simulink model "propagatorN"  (R2019b)
settings: Solver=ode113  StartTime=0.0  StopTime=86400  MaxStep=0.05  MinStep=1e-4  RelTol=1e-3  AbsTol=1e-13
values from neighbouring files (symbols this model uses):
  C = zeros(lmax,lmax)    [INIT.m]    (also in trajGen.m)
  J = zeros(lmax,1)    [INIT.m]    (also in trajGen.m)
  mi = 398600.435507    [INIT.m]    (also in trajGen.m)
  Rp = 6371    [INIT.m]    (also in trajGen.m)
  S = zeros(lmax,lmax)    [INIT.m]    (also in trajGen.m)
  X0 = [ R0 ; V0 ]    [INIT.m]    (also in trajGen.m)
settings Model: SimulationMode=rapid-accelerator  Creator=tomma  LastModifiedBy=antoniogenova

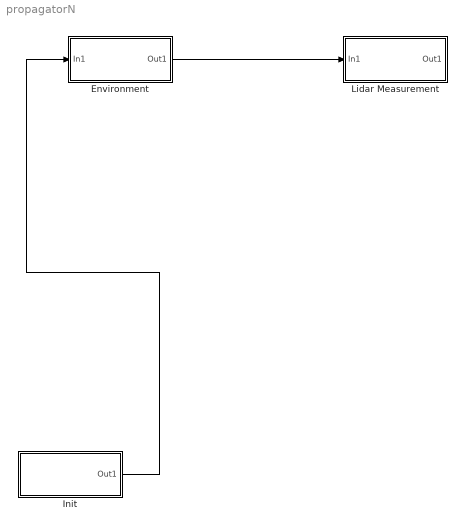
== system propagatorN ==
  "Environment " : Subsystem
  "Init " : Subsystem
  Lidar Measurement : Subsystem
  wires:
  "Init "/1(Out1) -> "Environment "/1(In1)
  "Environment "/1(Out1) -> Lidar Measurement/1(In1)

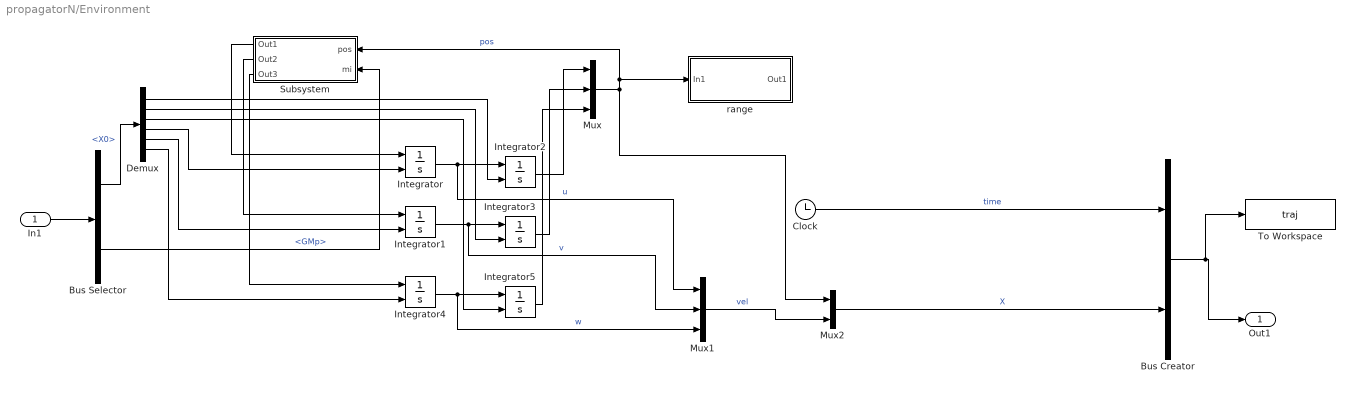
== system propagatorN/Environment  ==
  In1 : Inport
  Bus Creator : BusCreator  Inputs=2
  Bus Selector : BusSelector  OutputSignals=X0,GMp
  Clock : Clock
  Demux : Demux  Outputs=6
  Integrator{,1..5} (6 alike) : Integrator  InitialConditionSource=external  ContinuousStateAttributes="\"\""
  Mux : Mux  Inputs=3
  Mux1 : Mux  Inputs=3
  Mux2 : Mux  Inputs=2
  Subsystem : Subsystem
  To Workspace : ToWorkspace  VariableName=traj  SaveFormat=Timeseries  SampleTime=-1
  range : Subsystem
  Out1 : Outport
  wires:
  In1/1 -> Bus Selector/1
  Integrator4/1 -> Mux1/3, Integrator5/1  "w"
  Integrator1/1 -> Mux1/2, Integrator3/1  "v"
  Integrator/1 -> Mux1/1, Integrator2/1  "u"
  Bus Selector/1 -> Demux/1  "<X0>"
  Mux/1 -> Mux2/1, Subsystem/1(pos), range/1(In1)  "pos"
  Subsystem/1(Out1) -> Integrator/1
  Subsystem/2(Out2) -> Integrator1/1
  Subsystem/3(Out3) -> Integrator4/1
  Integrator2/1 -> Mux/1
  Integrator3/1 -> Mux/2
  Integrator5/1 -> Mux/3
  Mux1/1 -> Mux2/2  "vel"
  Bus Creator/1 -> To Workspace/1, Out1/1
  Bus Selector/2 -> Subsystem/2(mi)  "<GMp>"
  Demux/2 -> Integrator3/2
  Demux/1 -> Integrator2/2
  Demux/3 -> Integrator5/2
  Demux/4 -> Integrator/2
  Demux/5 -> Integrator1/2
  Demux/6 -> Integrator4/2
  Clock/1 -> Bus Creator/1  "time"
  Mux2/1 -> Bus Creator/2  "X"

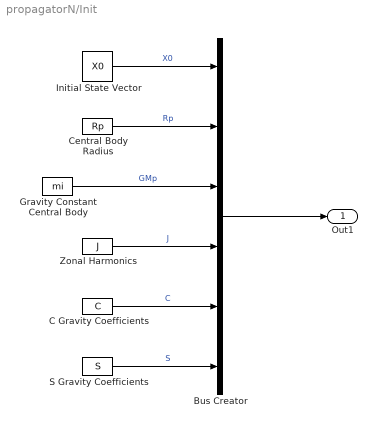
== system propagatorN/Init  ==
  Bus Creator : BusCreator  Inputs=6
  C Gravity Coefficients : Constant  Value=C
  Central Body Radius : Constant  Value=Rp
  Gravity Constant Central Body : Constant  Value=mi
  Initial State Vector : Constant  Value=X0
  S Gravity Coefficients : Constant  Value=S
  Zonal Harmonics : Constant  Value=J
  Out1 : Outport
  wires:
  Bus Creator/1 -> Out1/1
  Gravity Constant Central Body/1 -> Bus Creator/3  "GMp"
  Central Body Radius/1 -> Bus Creator/2  "Rp"
  Zonal Harmonics/1 -> Bus Creator/4  "J"
  C Gravity Coefficients/1 -> Bus Creator/5  "C"
  S Gravity Coefficients/1 -> Bus Creator/6  "S"
  Initial State Vector/1 -> Bus Creator/1  "X0"

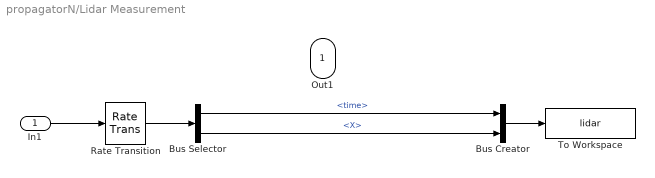
== system propagatorN/Lidar Measurement ==
  In1 : Inport
  Bus Creator : BusCreator  Inputs=2
  Bus Selector : BusSelector  OutputSignals=time,X
  Rate Transition : RateTransition  OutPortSampleTime=0.1
  To Workspace : ToWorkspace  VariableName=lidar  SaveFormat=Timeseries  SampleTime=-1
  Out1 : Outport
  wires:
  In1/1 -> Rate Transition/1
  Bus Selector/2 -> Bus Creator/2  "<X>"
  Bus Selector/1 -> Bus Creator/1  "<time>"
  Bus Creator/1 -> To Workspace/1
  Rate Transition/1 -> Bus Selector/1

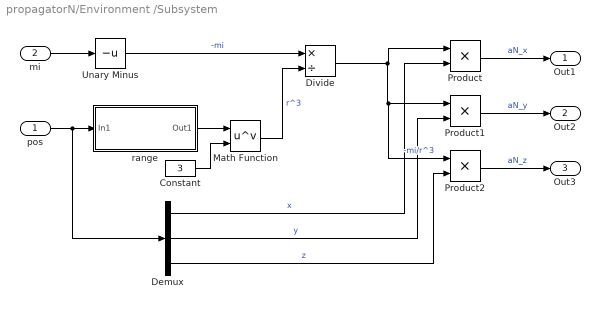
== system propagatorN/Environment /Subsystem ==
  pos : Inport
  mi : Inport  Port=2
  Constant : Constant  Value=3
  Demux : Demux  Outputs=3
  Divide : Product  Inputs=*/
  Math Function : Math  Operator=pow  SignedPower=off  SaturateOnIntegerOverflow=on
  Product : Product
  Product1 : Product
  Product2 : Product
  Unary Minus : UnaryMinus
  range : Subsystem
  Out1 : Outport
  Out2 : Outport  Port=2
  Out3 : Outport  Port=3
  wires:
  pos/1 -> Demux/1, range/1(In1)
  mi/1 -> Unary Minus/1
  Unary Minus/1 -> Divide/1  "-mi"
  Constant/1 -> Math Function/2
  range/1(Out1) -> Math Function/1
  Math Function/1 -> Divide/2  "r^3"
  Divide/1 -> Product2/1, Product1/1, Product/1  "-mi/r^3"
  Demux/1 -> Product/2  "x"
  Demux/2 -> Product1/2  "y"
  Demux/3 -> Product2/2  "z"
  Product/1 -> Out1/1  "aN_x"
  Product1/1 -> Out2/1  "aN_y"
  Product2/1 -> Out3/1  "aN_z"

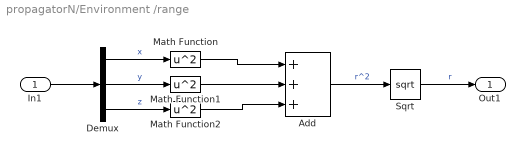
== system propagatorN/Environment /range ==
  In1 : Inport
  Add : Sum  Inputs=+++
  Demux : Demux  Outputs=3
  Math Function : Math  Operator=square  SignedPower=off  SaturateOnIntegerOverflow=on
  Math Function1 : Math  Operator=square  SignedPower=off  SaturateOnIntegerOverflow=on
  Math Function2 : Math  Operator=square  SignedPower=off  SaturateOnIntegerOverflow=on
  Sqrt : Sqrt  SaturateOnIntegerOverflow=on
  Out1 : Outport
  wires:
  In1/1 -> Demux/1
  Demux/1 -> Math Function/1  "x"
  Demux/2 -> Math Function1/1  "y"
  Demux/3 -> Math Function2/1  "z"
  Math Function/1 -> Add/1
  Math Function1/1 -> Add/2
  Math Function2/1 -> Add/3
  Add/1 -> Sqrt/1  "r^2"
  Sqrt/1 -> Out1/1  "r"

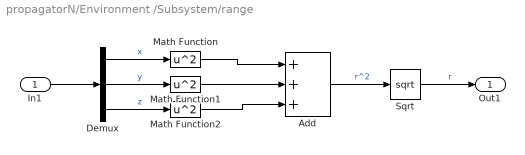
== system propagatorN/Environment /Subsystem/range ==
  In1 : Inport
  Add : Sum  Inputs=+++
  Demux : Demux  Outputs=3
  Math Function : Math  Operator=square  SignedPower=off  SaturateOnIntegerOverflow=on
  Math Function1 : Math  Operator=square  SignedPower=off  SaturateOnIntegerOverflow=on
  Math Function2 : Math  Operator=square  SignedPower=off  SaturateOnIntegerOverflow=on
  Sqrt : Sqrt  SaturateOnIntegerOverflow=on
  Out1 : Outport
  wires:
  In1/1 -> Demux/1
  Demux/1 -> Math Function/1  "x"
  Demux/2 -> Math Function1/1  "y"
  Demux/3 -> Math Function2/1  "z"
  Math Function/1 -> Add/1
  Math Function1/1 -> Add/2
  Math Function2/1 -> Add/3
  Add/1 -> Sqrt/1  "r^2"
  Sqrt/1 -> Out1/1  "r"
